simulink model "problema3"  (R2021a)
settings: Solver=VariableStepAuto  StartTime=0.0  StopTime=10.0  RelTol=1e-3
libraries: dspadpt3 x2
settings Model: Creator=Irek  LastModifiedBy=Irek

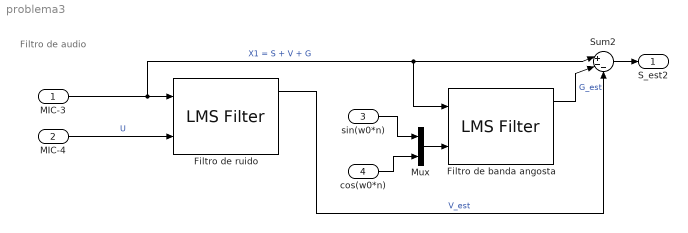
== system problema3 ==
  note: Filtro de audio
  MIC-3 : Inport
  MIC-4 : Inport  Port=2
  sin(w0*n) : Inport  Port=3
  cos(w0*n) : Inport  Port=4
  Filtro de banda angosta : dspadpt3/LMS Filter  Algo=LMS  L=32  stepflag=Dialog  mu=0.1  leakage=1.0  ic=0  Adapt=off  resetflag=None  weights=on  addnparflag=off  roundingMode=Floor  overflowMode=off  secondCoeffMode=Binary point scaling  secondCoeffWordLength=2  secondCoeffFracLength=15  prodOutput2Mode=Binary point scaling  prodOutput2FracLength=20  prodOutput3Mode=Binary point scaling  prodOutput3FracLength=20  prodOutput4Mode=Binary point scaling  prodOutput4FracLength=20  quotientMode=Binary point scaling  quotientFracLength=20  accum2Mode=Binary point scaling  accum2FracLength=20
      settings: SourceProductBaseCode=DS
  Filtro de ruido : dspadpt3/LMS Filter  Algo=LMS  L=32  stepflag=Dialog  mu=0.1  leakage=1.0  ic=0  Adapt=off  resetflag=None  weights=on  addnparflag=off  roundingMode=Floor  overflowMode=off  secondCoeffMode=Binary point scaling  secondCoeffWordLength=2  secondCoeffFracLength=15  prodOutput2Mode=Binary point scaling  prodOutput2FracLength=20  prodOutput3Mode=Binary point scaling  prodOutput3FracLength=20  prodOutput4Mode=Binary point scaling  prodOutput4FracLength=20  quotientMode=Binary point scaling  quotientFracLength=20  accum2Mode=Binary point scaling  accum2FracLength=20
      settings: SourceProductBaseCode=DS
  Mux : Mux  Inputs=2
  Sum2 : Sum  Inputs=|+--
  S_est2 : Outport
  wires:
  MIC-3/1 -> Filtro de banda angosta/1, Sum2/1, Filtro de ruido/1  "X1 = S + V + G"
  MIC-4/1 -> Filtro de ruido/2  "U"
  Filtro de ruido/1 -> Sum2/3  "V_est"
  sin(w0*n)/1 -> Mux/1
  Sum2/1 -> S_est2/1
  Mux/1 -> Filtro de banda angosta/2
  Filtro de banda angosta/1 -> Sum2/2  "G_est"
  cos(w0*n)/1 -> Mux/2
